simulink model "week1_problem1"  (R2020b)
settings: Solver=VariableStepAuto  StartTime=0.0  StopTime=10.0  RelTol=1e-3
model workspace (MAT data in the model file):
  B1 = Simulink.Parameter
  B1.Value = 50
  B1.DataType = 'auto'
  B1.Dimensions = [1 1]
  K1 = Simulink.Parameter
  K1.Value = 50
  K1.DataType = 'auto'
  K1.Dimensions = [1 1]
  K12 = Simulink.Parameter
  K12.Value = 1
  K12.DataType = 'auto'
  K12.Dimensions = [1 1]
  M1 = Simulink.Parameter
  M1.Value = 100
  M1.DataType = 'auto'
  M1.Dimensions = [1 1]
  M2 = Simulink.Parameter
  M2.Value = 1
  M2.DataType = 'auto'
  M2.Dimensions = [1 1]
undefined symbols (not defined in the file): h2r
settings Model: Creator=gokul  LastModifiedBy=gokul

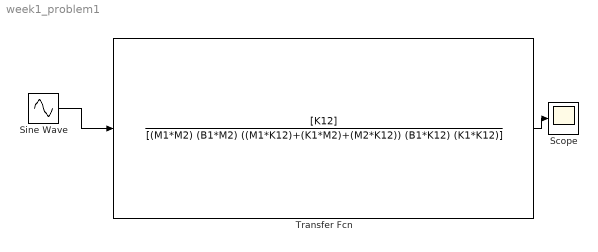
== system week1_problem1 ==
  Scope : Scope
  Sine Wave : Sin  Amplitude=2  Frequency=10 * h2r  SampleTime=0
  Transfer Fcn : TransferFcn  Numerator=[K12]  Denominator=[(M1*M2) (B1*M2) ((M1*K12)+(K1*M2)+(M2*K12)) (B1*K12) (K1*K12)]
  wires:
  Sine Wave/1 -> Transfer Fcn/1
  Transfer Fcn/1 -> Scope/1
